simulink library "QR_leg_rus_ver"  (R2021b)
settings: Solver=VariableStepAuto  StartTime=0.0  StopTime=10.0  RelTol=1e-3
values from neighbouring files (symbols this model uses):
  arm_inductance = 0.00025    [last_scores.mat]    (also in robotParameters.m)
  femur_mass = 0.888    [CostOfTransport.m]    (also in last_scores.mat; robotParameters.m)
  foot_mass = 0.06    [CostOfTransport.m]    (also in last_scores.mat; robotParameters.m)
  g_ratio = 1.5    [last_scores.mat]    (also in robotParameters.m = 3)
  k_d_fem = params(2)/10    [CostFcnPDcontroll.m]    (also in choice_ctrl_legs.m = 1; last_scores.mat = 1)
  k_d_tib = params(2)/10    [CostFcnPDcontroll.m]    (also in choice_ctrl_legs.m = 1; last_scores.mat = 1)
  k_i_fem = 0    [CostFcnPDcontroll.m]    (also in choice_ctrl_legs.m; last_scores.mat)
  k_i_tib = 0    [CostFcnPDcontroll.m]    (also in choice_ctrl_legs.m; last_scores.mat)
  k_p_fem = params(1)    [CostFcnPDcontroll.m]    (also in choice_ctrl_legs.m = 80; last_scores.mat = 80)
  k_p_tib = params(1)    [CostFcnPDcontroll.m]    (also in choice_ctrl_legs.m = 80; last_scores.mat = 80)
  m_voltage = 36    [last_scores.mat]    (also in robotParameters.m = 24)
  max_torque = 33.5    [last_scores.mat]    (also in robotParameters.m)
  N = (numel(params)-5)/4    [CostFuncOptimizeSpine.m]    (also in nonlinearContraints.m = (numel(x)-2)/4; nonlinearContraintsSpine.m = (numel(x)-5)/4; pampam.m = numel(params)/2)
  no_load_speed_motor = 21    [robotParameters.m]
  PWM_freq = 4000    [last_scores.mat]    (also in robotParameters.m = 100)
  rotor_damping = 0.09    [last_scores.mat]    (also in robotParameters.m)
  rotor_inertia = 7.2e-05    [last_scores.mat]    (also in robotParameters.m)
  stall_torque_motor = 33.5    [robotParameters.m]
  tibia_mass = 0.151    [CostOfTransport.m]    (also in last_scores.mat; robotParameters.m)
undefined symbols (not defined in the file or in its folder): AngleF, AngleT, motor_constant, OmegaF, OmegaT, TorqueF, TorqueT
libraries: fl_lib x18, nesl_utility x14, sm_lib x7, ee_lib x6
settings Model: Creator=boris_1863  LastModifiedBy=YEfim

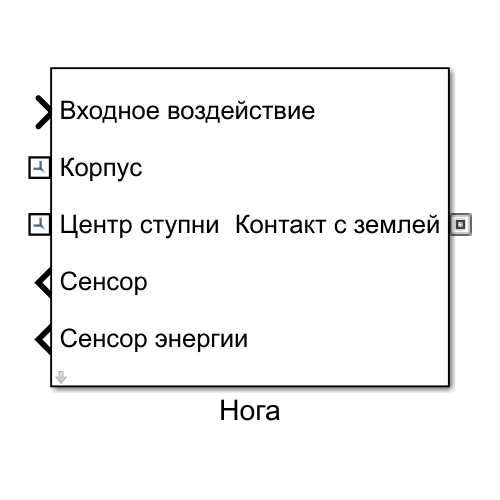
[thumbnail: Simulink's stored preview of the top-level diagram]
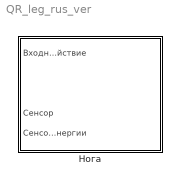
== system QR_leg_rus_ver ==
  Нога : Subsystem  mask{femur_l=0.13, tibia_l=0.18, leg_w=0.03, leg_w_t=0, qf_0=-135, qt_0=90, femur_cl=[0.2 0.2 1.0], tibia_cl=[0.6 0.6 1.0], kp_femur=k_p_fem, ki_femur=k_i_fem, kd_femur=k_d_fem, maxFemur=max_torque, minFemur=-max_torque, kp_tibia=k_p_tib, ki_tibia=k_i_tib, kd_tibia=k_d_tib, maxTibia=max_torque, minTibia=-max_torque, pwm_freq=PWM_freq, motor_voltage=m_voltage, motor_inductance=arm_inductance, motor_s_tau=stall_torque_motor, motor_nl_speed=no_load_speed_motor, motor_inertia=rotor_inertia, motor_damping=rotor_damping, gear_ratio=g_ratio}
      mask prompts: femur_l "Femur's length, [m]"; tibia_l "Tibia's length, [m]"; leg_w "Leg's width/height (fem), [m]"; leg_w_t "Leg's width/height (tib), [m]"; qf_0 "Initial angle for femur, [rad]"; qt_0 "Initial angle for tibia, [rad]"; femur_cl "Femur"; tibia_cl "Tibia"; kp_femur "coefficient prop"; ki_femur "coefficient int"; kd_femur "coefficient diff"; maxFemur "UpLimit"; minFemur "DownLimit"; kp_tibia "coefficient prop"; ki_tibia "coefficient int"; kd_tibia "coefficient diff"; maxTibia "UpLimit"; minTibia "DownLimit"; pwm_freq "PWM frequency [Hz]"; motor_voltage "Voltage amplitude [V]"; motor_inductance "Armeture inductance [H]"; motor_s_tau "Stall torque [H*m]"; motor_nl_speed "No-load speed [rad/s]"; motor_inertia "Rotor_inertia [kg*m^2]"; motor_damping "Rotor damping [N*m/(rad/s)]"; gear_ratio "Gear ratio"
      settings: PortSchema="{\"entries\":[{\"content\":{\"sides\":[{\"content\":{\"connectorIds\":[\"LConn1\"]},\"type\":\"ConnectorPlacement.EquallySpacedRectSide\",\"uuid\":\"ba4dde0f-eb28-4583-8625-c9de220f57e2\"},{\"content\":{\"connectorIds\":[\"In1\",\"RConn1\",\"RConn2\",\"Out1\",\"Out2\"],\"side\":\"RIGHT\"},\"type\":\"ConnectorPlacement.EquallySpacedRectSide\",\"uuid\":\"1870fe59-2a10-4ce1-bc4c-1177e0035dc8\"},{\"content\":{\"connectorIds\":[],\"side\":\"TOP\"},\"type\":\"ConnectorPlacement.EquallySpacedRectSide\",\"uuid\":\"23646215-7851-41ca-a2d9-d69aefcb7020\"}]},\"type\":\"ConnectorPlacement.EquallySpacedConnector\",\"uuid\":\"5f1753b4-5d27-4a38-a3ec-2c38d834fd8f\"}],\"packageUris\":[\"http://schema.mathworks.com/mf0/Connector/R2020b\"],\"version\":\"1.0\"}"
      mask DialogControl DescGroupVar Prompt: Leg's parameters
      mask DialogControl DescTextVar Prompt: Here we set parameters for a leg
      mask DialogControl ParameterGroupVar Prompt: Geometry
      mask DialogControl Container3 Prompt: Colours
      mask DialogControl Container7 Prompt: Control legs femur
      mask DialogControl Container5 Prompt: Control legs tibia
      mask DialogControl Container6 Prompt: Motor's model paramaters
      mask DialogControl Container8 Prompt: DC motor
      mask DialogControl Container12 Prompt: Electrical
      mask DialogControl Cont Prompt: Mechanical

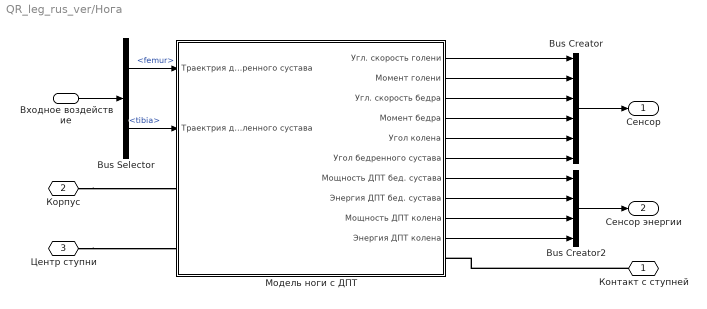
== system QR_leg_rus_ver/Нога ==
  Входное воздействие : Inport
  Bus Creator : BusCreator  Inputs=AngleF,AngleT,OmegaF,OmegaT,TorqueF,TorqueT
  Bus Creator2 : BusCreator  Inputs=4
  Bus Selector : BusSelector  OutputSignals=femur,tibia
  Модель ноги с ДПТ : Subsystem  AncestorBlock=QR_leg_rus_ver/Нога/Subsystem1/Motor  VariantControl=actuatorType == 1
  Контакт с ступней : PMIOPort  Side=Left
  Корпус : PMIOPort  Port=2  Side=Right
  Центр ступни : PMIOPort  Port=3  Side=Right
  Сенсор : Outport
  Сенсор энергии : Outport  Port=2
  wires:
  Входное воздействие/1 -> Bus Selector/1
  Bus Selector/1 -> Модель ноги с ДПТ/1(Траектрия движения бедренного сустава)  "<femur>"
  Bus Selector/2 -> Модель ноги с ДПТ/2(Траектрия движения коленного сустава)  "<tibia>"
  Bus Creator/1 -> Сенсор/1
  Bus Creator2/1 -> Сенсор энергии/1
  Модель ноги с ДПТ/7(Мощность ДПТ бед. сустава) -> Bus Creator2/1
  Модель ноги с ДПТ/8(Энергия ДПТ бед. сустава) -> Bus Creator2/2
  Модель ноги с ДПТ/9(Мощность ДПТ колена) -> Bus Creator2/3
  Модель ноги с ДПТ/10(Энергия ДПТ колена) -> Bus Creator2/4
  Модель ноги с ДПТ/1(Угл. скорость голени) -> Bus Creator/1
  Модель ноги с ДПТ/2(Момент голени) -> Bus Creator/2
  Модель ноги с ДПТ/3(Угл. скорость бедра) -> Bus Creator/3
  Модель ноги с ДПТ/4("Момент бедра ") -> Bus Creator/4
  Модель ноги с ДПТ/5(Угол колена) -> Bus Creator/5
  Модель ноги с ДПТ/6(Угол бедренного сустава) -> Bus Creator/6
  connections:
  Корпус/RConn1 -- Модель ноги с ДПТ/LConn1
  Контакт с ступней/RConn1 -- Модель ноги с ДПТ/RConn1
  Центр ступни/RConn1 -- Модель ноги с ДПТ/LConn2

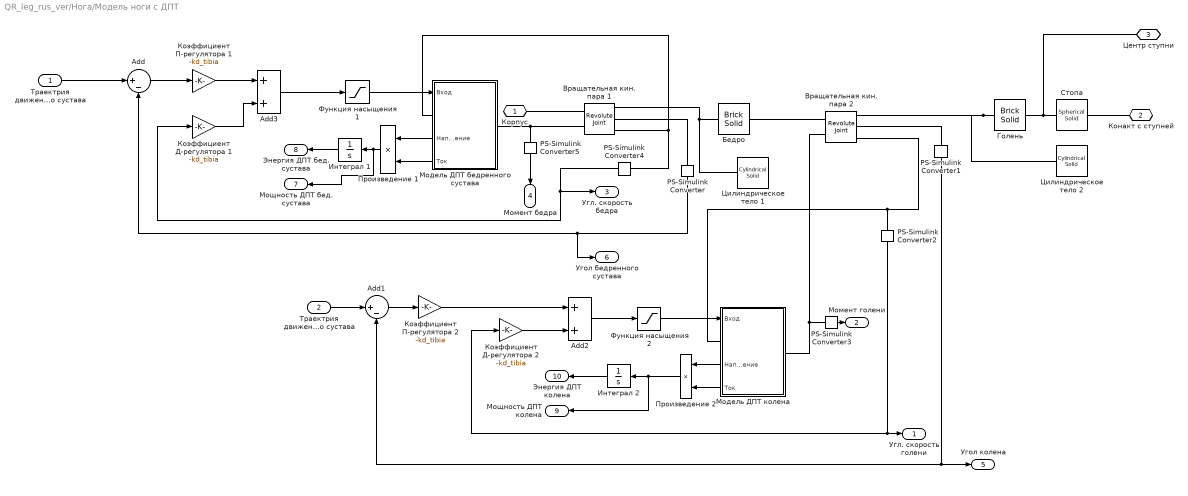
== system QR_leg_rus_ver/Нога/Модель ноги с ДПТ ==
  Траектрия движения бедренного сустава : Inport
  Траектрия движения коленного сустава : Inport  Port=2
  Add : Sum  Inputs=|+-
  Add1 : Sum  Inputs=|+-
  Add2 : Sum
  Add3 : Sum
  PS-Simulink Converter : nesl_utility/PS-Simulink Converter  PhysicalDomain=network_engine_domain  SubClassName=ps_output  LeftPortType=input  RightPortType=output  PseudoPeriodic=off  Frequencies=[]  Unit=inherit  AffineConversion=off
      settings: SourceProductBaseCode=PW,SS
  PS-Simulink Converter1 : nesl_utility/PS-Simulink Converter  PhysicalDomain=network_engine_domain  SubClassName=ps_output  LeftPortType=input  RightPortType=output  PseudoPeriodic=off  Frequencies=[]  Unit=rad  AffineConversion=off
      settings: SourceProductBaseCode=PW,SS
  PS-Simulink Converter2 : nesl_utility/PS-Simulink Converter  PhysicalDomain=network_engine_domain  SubClassName=ps_output  LeftPortType=input  RightPortType=output  PseudoPeriodic=off  Frequencies=[]  Unit=rad/s  AffineConversion=off
      settings: SourceProductBaseCode=PW,SS
  PS-Simulink Converter3 : nesl_utility/PS-Simulink Converter  PhysicalDomain=network_engine_domain  SubClassName=ps_output  LeftPortType=input  RightPortType=output  PseudoPeriodic=off  Frequencies=[]  Unit=N*m  AffineConversion=off
      settings: SourceProductBaseCode=PW,SS
  PS-Simulink Converter4 : nesl_utility/PS-Simulink Converter  PhysicalDomain=network_engine_domain  SubClassName=ps_output  LeftPortType=input  RightPortType=output  PseudoPeriodic=off  Frequencies=[]  Unit=rad/s  AffineConversion=off
      settings: SourceProductBaseCode=PW,SS
  PS-Simulink Converter5 : nesl_utility/PS-Simulink Converter  PhysicalDomain=network_engine_domain  SubClassName=ps_output  LeftPortType=input  RightPortType=output  PseudoPeriodic=off  Frequencies=[]  Unit=N*m  AffineConversion=off
      settings: SourceProductBaseCode=PW,SS
  Бедро : sm_lib/Body Elements/Brick Solid  GraphicAmbientColor=[0.15 0.15 0.15 1.0]  BasedOnType=Density  BrickDimensions=[femur_l leg_w(1) leg_w(2)]  BrickDimensionUnits=m  CenterOfMass=[0 0 0]  CenterOfMassUnits=m  GraphicDiffuseColor=femur_cl  Density=1000  DensityUnits=kg/m^3  DoExposeReferenceFrame=off  GraphicEmissiveColor=[0.0 0.0 0.0 1.0]  ExportEntireGeometry=off  SerializedFrames=<Frames><Frame><Id>Frame1</Id><Value><Name>F1</Name><Origin><Source>GeometricFeature</Source><FeatureName>-x surface</FeatureName></Origin><PrimaryAxis><DefinedDirection>+Z</DefinedDirection><Source>ReferenceFrame</Source><SourceDirection>+Z</SourceDirection><FeatureName></FeatureName></PrimaryAxis><SecondaryAxis><DefinedDirection>+X</DefinedDirection><Source>ReferenceFrame</Source><SourceDirection>+X</SourceDirection><FeatureName></FeatureName></SecondaryAxis></Value></Frame><Frame><Id>Frame2</Id><Value><Name>F2</Name><Origin><Source>GeometricFeature</Source><FeatureName>+x surface</FeatureName></Origin><PrimaryAxis><DefinedDirection>+Z</DefinedDirection><Source>ReferenceFrame</Source><SourceDirection>+Z</SourceDirection><FeatureName></FeatureName></PrimaryAxis><SecondaryAxis><DefinedDirection>+X</DefinedDirection><Source>ReferenceFrame</Source><SourceDirection>+X</SourceDirection><FeatureName></FeatureName></SecondaryAxis></Value></Frame></Frames>  MarkerShape=Sphere  MarkerSize=10  GraphicType=FromGeometry  InertiaType=PointMass  Mass=femur_mass  MassUnits=kg  MomentsOfInertia=[1 1 1]  MomentsOfInertiaUnits=kg*m^2  GraphicOpacity=1.0  ProductsOfInertia=[0 0 0]  ProductsOfInertiaUnits=kg*m^2  GraphicShininess=75  GraphicSpecularColor=[0.5 0.5 0.5 1.0]  GraphicVisPropType=SimpleVisualProperties
  Вращательная кин. пара 1 : sm_lib/Joints/Revolute Joint  JointMode=Normal  SenseConstraintForce=off  SenseConstraintForceX=off  SenseConstraintForceY=off  SenseConstraintForceZ=off  SenseConstraintTorque=off  SenseConstraintTorqueX=off  SenseConstraintTorqueY=off  SenseConstraintTorqueZ=off  SenseTotalForce=off  SenseTotalForceX=off  SenseTotalForceY=off  SenseTotalForceZ=off  SenseTotalTorque=off  SenseTotalTorqueX=off  SenseTotalTorqueY=off  SenseTotalTorqueZ=off  CompositeWrenchDir=FollowerOnBase  CompositeWrenchFrame=BaseFrame  EquilibriumPosition=0  EquilibriumPositionUnits=deg  SpringStiffness=0  SpringStiffnessUnits=N*m/deg  DampingCoefficient=0  DampingCoefficientUnits=N*m/(deg/s)  TorqueActuationMode=InputTorque  MotionActuationMode=ComputedMotion  SensePosition=on  SenseVelocity=on  SenseAcceleration=off  SenseTorqueForce=off  SenseLowerLimitTorqueForce=off  SenseUpperLimitTorqueForce=off  LowerLimitSpecify=off  LowerLimitBound=-90  LowerLimitBoundUnits=deg  LowerLimitStiffness=1e4  LowerLimitStiffnessUnits=N*m/deg  LowerLimitDamping=10  LowerLimitDampingUnits=N*m/(deg/s)  LowerLimitTransitionRegionWidth=0.1  LowerLimitTransitionRegionWidthUnits=deg  UpperLimitSpecify=off  UpperLimitBound=90  UpperLimitBoundUnits=deg  UpperLimitStiffness=1e4  UpperLimitStiffnessUnits=N*m/deg  UpperLimitDamping=10  UpperLimitDampingUnits=N*m/(deg/s)  UpperLimitTransitionRegionWidth=0.1  UpperLimitTransitionRegionWidthUnits=deg  PositionTargetSpecify=on  PositionTargetPriority=High  PositionTargetValue=qf_0  PositionTargetValueUnits=rad  VelocityTargetSpecify=off  VelocityTargetPriority=High  VelocityTargetValue=0  VelocityTargetValueUnits=deg/s
  Вращательная кин. пара 2 : sm_lib/Joints/Revolute Joint  JointMode=Normal  SenseConstraintForce=off  SenseConstraintForceX=off  SenseConstraintForceY=off  SenseConstraintForceZ=off  SenseConstraintTorque=off  SenseConstraintTorqueX=off  SenseConstraintTorqueY=off  SenseConstraintTorqueZ=off  SenseTotalForce=off  SenseTotalForceX=off  SenseTotalForceY=off  SenseTotalForceZ=off  SenseTotalTorque=off  SenseTotalTorqueX=off  SenseTotalTorqueY=off  SenseTotalTorqueZ=off  CompositeWrenchDir=FollowerOnBase  CompositeWrenchFrame=BaseFrame  EquilibriumPosition=0  EquilibriumPositionUnits=deg  SpringStiffness=0  SpringStiffnessUnits=N*m/deg  DampingCoefficient=0  DampingCoefficientUnits=N*m/(deg/s)  TorqueActuationMode=InputTorque  MotionActuationMode=ComputedMotion  SensePosition=on  SenseVelocity=on  SenseAcceleration=off  SenseTorqueForce=off  SenseLowerLimitTorqueForce=off  SenseUpperLimitTorqueForce=off  LowerLimitSpecify=off  LowerLimitBound=-90  LowerLimitBoundUnits=deg  LowerLimitStiffness=1e4  LowerLimitStiffnessUnits=N*m/deg  LowerLimitDamping=10  LowerLimitDampingUnits=N*m/(deg/s)  LowerLimitTransitionRegionWidth=0.1  LowerLimitTransitionRegionWidthUnits=deg  UpperLimitSpecify=off  UpperLimitBound=90  UpperLimitBoundUnits=deg  UpperLimitStiffness=1e4  UpperLimitStiffnessUnits=N*m/deg  UpperLimitDamping=10  UpperLimitDampingUnits=N*m/(deg/s)  UpperLimitTransitionRegionWidth=0.1  UpperLimitTransitionRegionWidthUnits=deg  PositionTargetSpecify=on  PositionTargetPriority=High  PositionTargetValue=qt_0  PositionTargetValueUnits=rad  VelocityTargetSpecify=off  VelocityTargetPriority=High  VelocityTargetValue=0  VelocityTargetValueUnits=deg/s
  Голень : sm_lib/Body Elements/Brick Solid  GraphicAmbientColor=[0.15 0.15 0.15 1.0]  BasedOnType=Density  BrickDimensions=[tibia_l leg_w_t(1) leg_w_t(2)]  BrickDimensionUnits=m  CenterOfMass=[0 0 0]  CenterOfMassUnits=m  GraphicDiffuseColor=tibia_cl  Density=1000  DensityUnits=kg/m^3  DoExposeReferenceFrame=off  GraphicEmissiveColor=[0.0 0.0 0.0 1.0]  ExportEntireGeometry=off  SerializedFrames=<Frames><Frame><Id>Frame1</Id><Value><Name>F1</Name><Origin><Source>GeometricFeature</Source><FeatureName>-x surface</FeatureName></Origin><PrimaryAxis><DefinedDirection>+Z</DefinedDirection><Source>ReferenceFrame</Source><SourceDirection>+Z</SourceDirection><FeatureName></FeatureName></PrimaryAxis><SecondaryAxis><DefinedDirection>+X</DefinedDirection><Source>ReferenceFrame</Source><SourceDirection>+X</SourceDirection><FeatureName></FeatureName></SecondaryAxis></Value></Frame><Frame><Id>Frame2</Id><Value><Name>F2</Name><Origin><Source>GeometricFeature</Source><FeatureName>+x surface</FeatureName></Origin><PrimaryAxis><DefinedDirection>+Z</DefinedDirection><Source>ReferenceFrame</Source><SourceDirection>+Z</SourceDirection><FeatureName></FeatureName></PrimaryAxis><SecondaryAxis><DefinedDirection>+X</DefinedDirection><Source>ReferenceFrame</Source><SourceDirection>+X</SourceDirection><FeatureName></FeatureName></SecondaryAxis></Value></Frame></Frames>  MarkerShape=Sphere  MarkerSize=10  GraphicType=FromGeometry  InertiaType=PointMass  Mass=tibia_mass  MassUnits=kg  MomentsOfInertia=[1 1 1]  MomentsOfInertiaUnits=kg*m^2  GraphicOpacity=1.0  ProductsOfInertia=[0 0 0]  ProductsOfInertiaUnits=kg*m^2  GraphicShininess=75  GraphicSpecularColor=[0.5 0.5 0.5 1.0]  GraphicVisPropType=SimpleVisualProperties
  Интеграл 1 : Integrator
  Интеграл 2 : Integrator
  Коэффициент Д-регулятора 1 : Gain  Gain=-kd_tibia
  Коэффициент Д-регулятора 2 : Gain  Gain=-kd_tibia
  Коэффициент П-регулятора 1 : Gain  Gain=-kd_tibia
  Коэффициент П-регулятора 2 : Gain  Gain=-kd_tibia
  Модель ДПТ бедренного сустава : Subsystem  AncestorBlock=QR_leg_rus_ver/Нога/Subsystem1/Motor/Motor Model T  VariantControl=Choice
      settings: PortSchema="{\"entries\":[{\"content\":{\"sides\":[{\"content\":{\"connectorIds\":[\"LConn1\"]},\"type\":\"ConnectorPlacement.EquallySpacedRectSide\",\"uuid\":\"8cbf5340-af4d-433b-8c30-eaee76423689\"},{\"content\":{\"connectorIds\":[\"In1\",\"RConn1\",\"Out1\",\"Out2\"],\"side\":\"RIGHT\"},\"type\":\"ConnectorPlacement.EquallySpacedRectSide\",\"uuid\":\"3d9d5440-8031-4c97-81de-c93cb50b20e1\"},{\"content\":{\"connectorIds\":[],\"side\":\"TOP\"},\"type\":\"ConnectorPlacement.EquallySpacedRectSide\",\"uuid\":\"6dede49e-1776-42b7-ab91-8c4960b52fc7\"}]},\"type\":\"ConnectorPlacement.EquallySpacedConnector\",\"uuid\":\"ecb595c5-898e-4247-93ce-92177f9e6279\"}],\"packageUris\":[\"http://schema.mathworks.com/mf0/Connector/R2020b\"],\"version\":\"1.0\"}"
  Модель ДПТ колена : Subsystem  VariantControl=Choice
      settings: PortSchema="{\"entries\":[{\"content\":{\"sides\":[{\"content\":{\"connectorIds\":[\"LConn1\"]},\"type\":\"ConnectorPlacement.EquallySpacedRectSide\",\"uuid\":\"8cbf5340-af4d-433b-8c30-eaee76423689\"},{\"content\":{\"connectorIds\":[\"In1\",\"RConn1\",\"Out1\",\"Out2\"],\"side\":\"RIGHT\"},\"type\":\"ConnectorPlacement.EquallySpacedRectSide\",\"uuid\":\"3d9d5440-8031-4c97-81de-c93cb50b20e1\"},{\"content\":{\"connectorIds\":[],\"side\":\"TOP\"},\"type\":\"ConnectorPlacement.EquallySpacedRectSide\",\"uuid\":\"6dede49e-1776-42b7-ab91-8c4960b52fc7\"}]},\"type\":\"ConnectorPlacement.EquallySpacedConnector\",\"uuid\":\"ecb595c5-898e-4247-93ce-92177f9e6279\"}],\"packageUris\":[\"http://schema.mathworks.com/mf0/Connector/R2020b\"],\"version\":\"1.0\"}"
  Произведение 1 : Product
  Произведение 2 : Product
  Стопа : sm_lib/Body Elements/Spherical Solid  GraphicAmbientColor=[0.15 0.15 0.15 1.0]  BasedOnType=Density  CenterOfMass=[0 0 0]  CenterOfMassUnits=m  GraphicDiffuseColor=tibia_cl  Density=1000  DensityUnits=kg/m^3  DoExposeReferenceFrame=on  GraphicEmissiveColor=[0.0 0.0 0.0 1.0]  ExportEntireGeometry=on  SerializedExposedGeometries=<ExposedGeometries><ExposedGeometry><RawGeometryId>entire</RawGeometryId><ExposedGeometryId>G</ExposedGeometryId></ExposedGeometry></ExposedGeometries>  SerializedFrames=<Frames/>  MarkerShape=Sphere  MarkerSize=10  GraphicType=FromGeometry  InertiaType=PointMass  Mass=foot_mass  MassUnits=kg  MomentsOfInertia=[1 1 1]  MomentsOfInertiaUnits=kg*m^2  GraphicOpacity=1.0  ProductsOfInertia=[0 0 0]  ProductsOfInertiaUnits=kg*m^2  GraphicShininess=75  GraphicSpecularColor=[0.5 0.5 0.5 1.0]  SphereRadius=sp_rad  SphereRadiusUnits=m  GraphicVisPropType=SimpleVisualProperties
  Функция насыщения 1 : Saturate  UpperLimit=max_torque  LowerLimit=-max_torque
  Функция насыщения 2 : Saturate  UpperLimit=max_torque  LowerLimit=-max_torque
  Цилиндрическое тело 1 : sm_lib/Body Elements/Cylindrical Solid  GraphicAmbientColor=[0.15 0.15 0.15 1.0]  BasedOnType=Density  CenterOfMass=[0 0 0]  CenterOfMassUnits=m  GraphicDiffuseColor=femur_cl  CylinderLength=leg_w(2)  CylinderLengthUnits=m  CylinderRadius=leg_w(1)/2  CylinderRadiusUnits=m  Density=0  DensityUnits=kg/m^3  DoExposeReferenceFrame=on  GraphicEmissiveColor=[0.0 0.0 0.0 1.0]  ExportEntireGeometry=off  SerializedFrames=<Frames/>  MarkerShape=Sphere  MarkerSize=10  GraphicType=FromGeometry  InertiaType=CalculateFromGeometry  Mass=1  MassUnits=kg  MomentsOfInertia=[1 1 1]  MomentsOfInertiaUnits=kg*m^2  GraphicOpacity=1.0  ProductsOfInertia=[0 0 0]  ProductsOfInertiaUnits=kg*m^2  GraphicShininess=75  GraphicSpecularColor=[0.5 0.5 0.5 1.0]  GraphicVisPropType=SimpleVisualProperties
  Цилиндрическое тело 2 : sm_lib/Body Elements/Cylindrical Solid  GraphicAmbientColor=[0.15 0.15 0.15 1.0]  BasedOnType=Density  CenterOfMass=[0 0 0]  CenterOfMassUnits=m  GraphicDiffuseColor=femur_cl  CylinderLength=leg_w(2)  CylinderLengthUnits=m  CylinderRadius=leg_w(1)/2  CylinderRadiusUnits=m  Density=0  DensityUnits=kg/m^3  DoExposeReferenceFrame=on  GraphicEmissiveColor=[0.0 0.0 0.0 1.0]  ExportEntireGeometry=off  SerializedFrames=<Frames/>  MarkerShape=Sphere  MarkerSize=10  GraphicType=FromGeometry  InertiaType=CalculateFromGeometry  Mass=1  MassUnits=kg  MomentsOfInertia=[1 1 1]  MomentsOfInertiaUnits=kg*m^2  GraphicOpacity=1.0  ProductsOfInertia=[0 0 0]  ProductsOfInertiaUnits=kg*m^2  GraphicShininess=75  GraphicSpecularColor=[0.5 0.5 0.5 1.0]  GraphicVisPropType=SimpleVisualProperties
  Корпус : PMIOPort  Side=Left
  Конакт с ступней : PMIOPort  Port=2  Side=Right
  Центр ступни : PMIOPort  Port=3  Side=Left
  Угл. скорость голени : Outport
  Момент голени : Outport  Port=2
  Угл. скорость бедра : Outport  Port=3
  "Момент бедра " : Outport  Port=4
  Угол колена : Outport  Port=5
  Угол бедренного сустава : Outport  Port=6
  Мощность ДПТ бед. сустава : Outport  Port=7
  Энергия ДПТ бед. сустава : Outport  Port=8
  Мощность ДПТ колена : Outport  Port=9
  Энергия ДПТ колена : Outport  Port=10
  wires:
  PS-Simulink Converter5/1 -> "Момент бедра "/1
  PS-Simulink Converter3/1 -> Момент голени/1
  Траектрия движения бедренного сустава/1 -> Add/1
  PS-Simulink Converter4/1 -> Коэффициент Д-регулятора 1/1, Угл. скорость бедра/1
  Add/1 -> Коэффициент П-регулятора 1/1
  PS-Simulink Converter1/1 -> Угол колена/1, Add1/2
  PS-Simulink Converter2/1 -> Коэффициент Д-регулятора 2/1, Угл. скорость голени/1
  Add1/1 -> Коэффициент П-регулятора 2/1
  Траектрия движения коленного сустава/1 -> Add1/1
  Модель ДПТ колена/2(Ток) -> Произведение 2/2
  Модель ДПТ колена/1(Напряжение) -> Произведение 2/1
  Модель ДПТ бедренного сустава/1(Напряжение) -> Произведение 1/1
  Модель ДПТ бедренного сустава/2(Ток) -> Произведение 1/2
  PS-Simulink Converter/1 -> Add/2, Угол бедренного сустава/1
  Коэффициент П-регулятора 1/1 -> Add3/1
  Коэффициент П-регулятора 2/1 -> Add2/1
  Add3/1 -> Функция насыщения 1/1
  Функция насыщения 1/1 -> Модель ДПТ бедренного сустава/1(Вход)
  Add2/1 -> Функция насыщения 2/1
  Функция насыщения 2/1 -> Модель ДПТ колена/1(Вход)
  Коэффициент Д-регулятора 2/1 -> Add2/2
  Произведение 1/1 -> Мощность ДПТ бед. сустава/1, Интеграл 1/1
  Интеграл 1/1 -> Энергия ДПТ бед. сустава/1
  Интеграл 2/1 -> Энергия ДПТ колена/1
  Произведение 2/1 -> Интеграл 2/1, Мощность ДПТ колена/1
  Коэффициент Д-регулятора 1/1 -> Add3/2
  connections:
  Бедро/LConn1 -- Цилиндрическое тело 1/RConn1 -- Вращательная кин. пара 1/RConn1
  Голень/LConn1 -- Вращательная кин. пара 2/RConn1 -- Цилиндрическое тело 2/RConn1
  PS-Simulink Converter4/LConn1 -- Модель ДПТ бедренного сустава/RConn1 -- Вращательная кин. пара 1/RConn3
  PS-Simulink Converter5/LConn1 -- Модель ДПТ бедренного сустава/LConn1 -- Вращательная кин. пара 1/LConn2
  PS-Simulink Converter3/LConn1 -- Модель ДПТ колена/LConn1 -- Вращательная кин. пара 2/LConn2
  Корпус/RConn1 -- Вращательная кин. пара 1/LConn1
  Вращательная кин. пара 2/RConn3 -- Модель ДПТ колена/RConn1 -- PS-Simulink Converter2/LConn1
  PS-Simulink Converter/LConn1 -- Вращательная кин. пара 1/RConn2
  Вращательная кин. пара 2/LConn1 -- Бедро/RConn1
  PS-Simulink Converter1/LConn1 -- Вращательная кин. пара 2/RConn2
  Конакт с ступней/RConn1 -- Стопа/LConn1
  Стопа/RConn1 -- Центр ступни/RConn1 -- Голень/RConn1

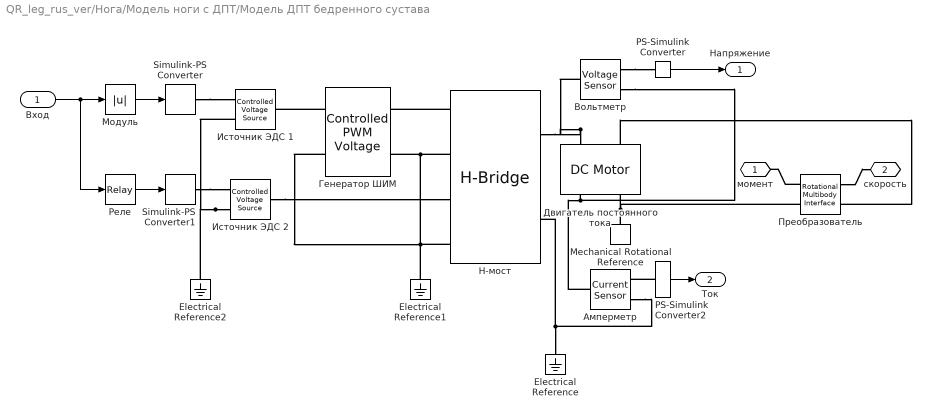
== system QR_leg_rus_ver/Нога/Модель ноги с ДПТ/Модель ДПТ бедренного сустава ==
  Вход : Inport
  Electrical Reference : fl_lib/Electrical/Electrical Elements/Electrical Reference
  Electrical Reference1 : fl_lib/Electrical/Electrical Elements/Electrical Reference
  Electrical Reference2 : fl_lib/Electrical/Electrical Elements/Electrical Reference
  H-мост : ee_lib/Semiconductors & Converters/Converters/H-Bridge  supply_ports=ee.enum.supply_ports.hidesupply  pwm_or_av=ee.enum.pwm_or_av.averaged  regenerative_braking_mode=ee.enum.converters.regenerative_braking_mode.always_enabled  discontinuous=ee.enum.current_profile.continuous  freewheeling_mode=ee.enum.converters.freewheeling_mode.one_switch_one_diode  Rload=10 Ohm  Lload=1e-5 H  F=10 kHz  Venable=motor_voltage/2 V  Vmax=motor_voltage V  Vreverse=0.5 V  Vbrake=0.5 V  Vm=motor_voltage V  Ron=1e-3 Ohm  Don=1e-3 Ohm  Goff=1e-6 S  Tmeas=298.15 K  Ron2=0.1 Ohm  Don2=0.05 Ohm  Tmeas2=398.15 K  thermal_mass=100 J/K  initial_temperature=298.15 K
  Mechanical Rotational Reference : fl_lib/Mechanical/Rotational Elements/Mechanical Rotational Reference
  PS-Simulink Converter : nesl_utility/PS-Simulink Converter  PhysicalDomain=network_engine_domain  SubClassName=ps_output  LeftPortType=input  RightPortType=output  PseudoPeriodic=off  Frequencies=[]  Unit=V  AffineConversion=off
      settings: SourceProductBaseCode=PW,SS
  PS-Simulink Converter2 : nesl_utility/PS-Simulink Converter  PhysicalDomain=network_engine_domain  SubClassName=ps_output  LeftPortType=input  RightPortType=output  PseudoPeriodic=off  Frequencies=[]  Unit=A  AffineConversion=off
      settings: SourceProductBaseCode=PW,SS
  Simulink-PS Converter : nesl_utility/Simulink-PS Converter  PhysicalDomain=network_engine_domain  SubClassName=ps_input  LeftPortType=input  RightPortType=output  PseudoPeriodic=off  Frequencies=[]  NoiseDistribution=none  NoiseParameters=[]  Unit=1  AffineConversion=off  FilteringAndDerivatives=provide  SimscapeFilterOrder=1  InputFilterTimeConstant=0.005  UdotUserProvided=0
  Simulink-PS Converter1 : nesl_utility/Simulink-PS Converter  PhysicalDomain=network_engine_domain  SubClassName=ps_input  LeftPortType=input  RightPortType=output  PseudoPeriodic=off  Frequencies=[]  NoiseDistribution=none  NoiseParameters=[]  Unit=1  AffineConversion=off  FilteringAndDerivatives=provide  SimscapeFilterOrder=1  InputFilterTimeConstant=0.005  UdotUserProvided=0
  Амперметр : fl_lib/Electrical/Electrical Sensors/Current Sensor
  Вольтметр : fl_lib/Electrical/Electrical Sensors/Voltage Sensor
  Генератор ШИМ : ee_lib/Integrated Circuits/Controlled PWM Voltage  F=pwm_freq Hz  TD=0 s  pulse_width_offset=0 s  pulse_min=0 s  pwm_or_av=2  event_type=1  sample_time=1e-6 s  Vmin=0 V  Vmax=max_torque V  Vm=motor_voltage V  u_min=0  u_max=1
  Двигатель постоянного тока : ee_lib/Electromechanical/Brushed Motors/DC Motor  field_option=ee.enum.field_option.pm  Rf=100 Ohm  Lf=1 H  Laf=0.15 H  If0=0 A  parameterization=ee.enum.dcparam_option.torque_speed  Ra=motor_resistance Ohm  La=motor_inductance H  emf_or_torque=ee.enum.emf_or_torque.ki  Kv=0.01 V/rpm  Ki=motor_constant N*m/A  T_stall=motor_s_tau N*m  w_max=motor_nl_speed rad/s  w_rated=1.5e+4 rpm  P_rated=0.08 W  V_rated=motor_voltage V  lam_param=ee.enum.lam_param.damping  i_noload=0 A  V_i_noload=1.5 V  J=motor_inertia kg*m^2  lam=motor_damping N*m/(rad/s)  speed0=0 rpm  enable_fault_armature=simscape.enum.onoff.off  rev_faulted=1 / 3  G_faulted_armature=1e-5 S  fault_trigger_armature=ee.enum.faults.faultTrigger.temporal  t_fault_armature=1 s  max_permissible_current_armature=inf A  t_fail_on_current_armature=1 s  enable_fault_field=simscape.enum.onoff.off  G_faulted_field=1e-5 S  fault_trigger_field=ee.enum.faults.faultTrigger.temporal  t_fault_field=1 s  max_permissible_current_field=inf A  t_fail_on_current_field=1 s  fault_action=simscape.enum.assert.action.none  alpha=3.93e-3 1/K  Tmeas=25 degC  thermal_mass=100 J/K  initial_temperature=25 degC
  Источник ЭДС 1 : fl_lib/Electrical/Electrical Sources/Controlled Voltage Source
  Источник ЭДС 2 : fl_lib/Electrical/Electrical Sources/Controlled Voltage Source
  Модуль : Abs  ZeroCross=off
  Преобразователь : fl_lib/Mechanical/Multibody Interfaces/Rotational Multibody Interface
      settings: SourceProductBaseCode=SS
  Реле : Relay  OnSwitchValue=1  OffSwitchValue=-1  OnOutputValue=0  OffOutputValue=1  ZeroCross=off
  момент : PMIOPort  Side=Left
  скорость : PMIOPort  Port=2  Side=Right
  Напряжение : Outport
  Ток : Outport  Port=2
  wires:
  PS-Simulink Converter2/1 -> Ток/1
  PS-Simulink Converter/1 -> Напряжение/1
  Модуль/1 -> Simulink-PS Converter/1
  Реле/1 -> Simulink-PS Converter1/1
  Вход/1 -> Модуль/1, Реле/1
  connections:
  Вольтметр/RConn1 -- PS-Simulink Converter/LConn1
  PS-Simulink Converter2/LConn1 -- Амперметр/RConn1
  Амперметр/RConn2 -- H-мост/RConn2 -- Electrical Reference/LConn1
  Вольтметр/RConn2 -- Амперметр/LConn1 -- Двигатель постоянного тока/RConn1
  Источник ЭДС 2/LConn1 -- H-мост/LConn3
  Simulink-PS Converter1/RConn1 -- Источник ЭДС 2/RConn1
  Двигатель постоянного тока/LConn1 -- Вольтметр/LConn1 -- H-мост/RConn1
  Двигатель постоянного тока/RConn2 -- Преобразователь/LConn2 -- Mechanical Rotational Reference/LConn1
  Simulink-PS Converter/RConn1 -- Источник ЭДС 1/RConn1
  Генератор ШИМ/LConn1 -- Источник ЭДС 1/LConn1
  Преобразователь/LConn1 -- момент/RConn1
  H-мост/LConn1 -- Генератор ШИМ/RConn1
  Источник ЭДС 2/RConn2 -- Источник ЭДС 1/RConn2 -- Electrical Reference2/LConn1
  Преобразователь/RConn1 -- скорость/RConn1
  H-мост/LConn4 -- Electrical Reference1/LConn1 -- Генератор ШИМ/LConn2 -- H-мост/LConn2 -- Генератор ШИМ/RConn2
  Двигатель постоянного тока/LConn2 -- Преобразователь/RConn2

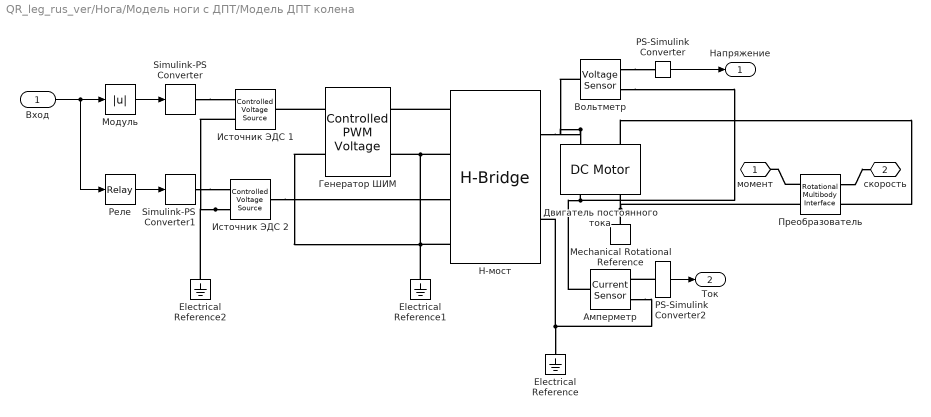
== system QR_leg_rus_ver/Нога/Модель ноги с ДПТ/Модель ДПТ колена ==
  Вход : Inport
  Electrical Reference : fl_lib/Electrical/Electrical Elements/Electrical Reference
  Electrical Reference1 : fl_lib/Electrical/Electrical Elements/Electrical Reference
  Electrical Reference2 : fl_lib/Electrical/Electrical Elements/Electrical Reference
  H-мост : ee_lib/Semiconductors & Converters/Converters/H-Bridge  supply_ports=ee.enum.supply_ports.hidesupply  pwm_or_av=ee.enum.pwm_or_av.averaged  regenerative_braking_mode=ee.enum.converters.regenerative_braking_mode.always_enabled  discontinuous=ee.enum.current_profile.continuous  freewheeling_mode=ee.enum.converters.freewheeling_mode.one_switch_one_diode  Rload=10 Ohm  Lload=1e-5 H  F=10 kHz  Venable=motor_voltage/2 V  Vmax=motor_voltage V  Vreverse=0.5 V  Vbrake=0.5 V  Vm=motor_voltage V  Ron=1e-3 Ohm  Don=1e-3 Ohm  Goff=1e-6 S  Tmeas=298.15 K  Ron2=0.1 Ohm  Don2=0.05 Ohm  Tmeas2=398.15 K  thermal_mass=100 J/K  initial_temperature=298.15 K
  Mechanical Rotational Reference : fl_lib/Mechanical/Rotational Elements/Mechanical Rotational Reference
  PS-Simulink Converter : nesl_utility/PS-Simulink Converter  PhysicalDomain=network_engine_domain  SubClassName=ps_output  LeftPortType=input  RightPortType=output  PseudoPeriodic=off  Frequencies=[]  Unit=V  AffineConversion=off
      settings: SourceProductBaseCode=PW,SS
  PS-Simulink Converter2 : nesl_utility/PS-Simulink Converter  PhysicalDomain=network_engine_domain  SubClassName=ps_output  LeftPortType=input  RightPortType=output  PseudoPeriodic=off  Frequencies=[]  Unit=A  AffineConversion=off
      settings: SourceProductBaseCode=PW,SS
  Simulink-PS Converter : nesl_utility/Simulink-PS Converter  PhysicalDomain=network_engine_domain  SubClassName=ps_input  LeftPortType=input  RightPortType=output  PseudoPeriodic=off  Frequencies=[]  NoiseDistribution=none  NoiseParameters=[]  Unit=1  AffineConversion=off  FilteringAndDerivatives=provide  SimscapeFilterOrder=1  InputFilterTimeConstant=0.005  UdotUserProvided=0
  Simulink-PS Converter1 : nesl_utility/Simulink-PS Converter  PhysicalDomain=network_engine_domain  SubClassName=ps_input  LeftPortType=input  RightPortType=output  PseudoPeriodic=off  Frequencies=[]  NoiseDistribution=none  NoiseParameters=[]  Unit=1  AffineConversion=off  FilteringAndDerivatives=provide  SimscapeFilterOrder=1  InputFilterTimeConstant=0.005  UdotUserProvided=0
  Амперметр : fl_lib/Electrical/Electrical Sensors/Current Sensor
  Вольтметр : fl_lib/Electrical/Electrical Sensors/Voltage Sensor
  Генератор ШИМ : ee_lib/Integrated Circuits/Controlled PWM Voltage  F=pwm_freq Hz  TD=0 s  pulse_width_offset=0 s  pulse_min=0 s  pwm_or_av=2  event_type=1  sample_time=1e-6 s  Vmin=0 V  Vmax=max_torque V  Vm=motor_voltage V  u_min=0  u_max=1
  Двигатель постоянного тока : ee_lib/Electromechanical/Brushed Motors/DC Motor  field_option=ee.enum.field_option.pm  Rf=100 Ohm  Lf=1 H  Laf=0.15 H  If0=0 A  parameterization=ee.enum.dcparam_option.torque_speed  Ra=motor_resistance Ohm  La=motor_inductance H  emf_or_torque=ee.enum.emf_or_torque.ki  Kv=0.01 V/rpm  Ki=motor_constant N*m/A  T_stall=motor_s_tau N*m  w_max=motor_nl_speed rad/s  w_rated=1.5e+4 rpm  P_rated=0.08 W  V_rated=motor_voltage V  lam_param=ee.enum.lam_param.damping  i_noload=0 A  V_i_noload=1.5 V  J=motor_inertia kg*m^2  lam=motor_damping N*m/(rad/s)  speed0=0 rpm  enable_fault_armature=simscape.enum.onoff.off  rev_faulted=1 / 3  G_faulted_armature=1e-5 S  fault_trigger_armature=ee.enum.faults.faultTrigger.temporal  t_fault_armature=1 s  max_permissible_current_armature=inf A  t_fail_on_current_armature=1 s  enable_fault_field=simscape.enum.onoff.off  G_faulted_field=1e-5 S  fault_trigger_field=ee.enum.faults.faultTrigger.temporal  t_fault_field=1 s  max_permissible_current_field=inf A  t_fail_on_current_field=1 s  fault_action=simscape.enum.assert.action.none  alpha=3.93e-3 1/K  Tmeas=25 degC  thermal_mass=100 J/K  initial_temperature=25 degC
  Источник ЭДС 1 : fl_lib/Electrical/Electrical Sources/Controlled Voltage Source
  Источник ЭДС 2 : fl_lib/Electrical/Electrical Sources/Controlled Voltage Source
  Модуль : Abs  ZeroCross=off
  Преобразователь : fl_lib/Mechanical/Multibody Interfaces/Rotational Multibody Interface
      settings: SourceProductBaseCode=SS
  Реле : Relay  OnSwitchValue=1  OffSwitchValue=-1  OnOutputValue=0  OffOutputValue=1  ZeroCross=off
  момент : PMIOPort  Side=Left
  скорость : PMIOPort  Port=2  Side=Right
  Напряжение : Outport
  Ток : Outport  Port=2
  wires:
  PS-Simulink Converter2/1 -> Ток/1
  PS-Simulink Converter/1 -> Напряжение/1
  Модуль/1 -> Simulink-PS Converter/1
  Реле/1 -> Simulink-PS Converter1/1
  Вход/1 -> Модуль/1, Реле/1
  connections:
  Вольтметр/RConn1 -- PS-Simulink Converter/LConn1
  PS-Simulink Converter2/LConn1 -- Амперметр/RConn1
  Амперметр/RConn2 -- H-мост/RConn2 -- Electrical Reference/LConn1
  Вольтметр/RConn2 -- Амперметр/LConn1 -- Двигатель постоянного тока/RConn1
  Источник ЭДС 2/LConn1 -- H-мост/LConn3
  Simulink-PS Converter1/RConn1 -- Источник ЭДС 2/RConn1
  Двигатель постоянного тока/LConn1 -- Вольтметр/LConn1 -- H-мост/RConn1
  Двигатель постоянного тока/RConn2 -- Преобразователь/LConn2 -- Mechanical Rotational Reference/LConn1
  Simulink-PS Converter/RConn1 -- Источник ЭДС 1/RConn1
  Генератор ШИМ/LConn1 -- Источник ЭДС 1/LConn1
  Преобразователь/LConn1 -- момент/RConn1
  H-мост/LConn1 -- Генератор ШИМ/RConn1
  Источник ЭДС 2/RConn2 -- Источник ЭДС 1/RConn2 -- Electrical Reference2/LConn1
  Преобразователь/RConn1 -- скорость/RConn1
  H-мост/LConn4 -- Electrical Reference1/LConn1 -- Генератор ШИМ/LConn2 -- H-мост/LConn2 -- Генератор ШИМ/RConn2
  Двигатель постоянного тока/LConn2 -- Преобразователь/RConn2
